simulink model "Prelab1a_simulink_starter"  (R2016a)
settings: Solver=FixedStepDiscrete  StartTime=0.0  StopTime=10.0  FixedStep=5e-3  RelTol=1e-3
settings Model: Creator=katiebyl  LastModifiedBy=katiebyl
settings RTWCC: BuildConfiguration=Faster Runs

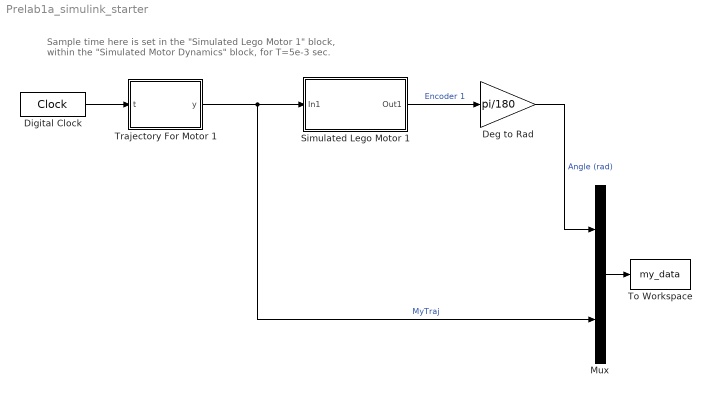
== system Prelab1a_simulink_starter ==
  note: Sample time here is set in the "Simulated Lego Motor 1" block,
      | within the "Simulated Motor Dynamics" block, for T=5e-3 sec.
  Deg to Rad : Gain  Gain=pi/180
  Digital Clock : DigitalClock  SampleTime=5e-3
  Mux : Mux  Inputs=2
  Simulated Lego Motor 1 : Subsystem
  To Workspace : ToWorkspace  VariableName=my_data  SaveFormat=Structure With Time  SampleTime=-1
  Trajectory For Motor 1 : MATLAB Function  TreatAsAtomicUnit=on
  wires:
  Simulated Lego Motor 1/1(Out1) -> Deg to Rad/1  "Encoder 1"
  Deg to Rad/1 -> Mux/1  "Angle (rad)"
  Mux/1 -> To Workspace/1
  Digital Clock/1 -> Trajectory For Motor 1/1(t)
  Trajectory For Motor 1/1(y) -> Mux/2, Simulated Lego Motor 1/1(In1)  "MyTraj"

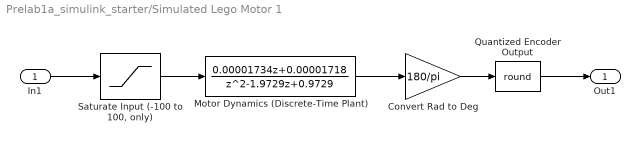
== system Prelab1a_simulink_starter/Simulated Lego Motor 1 ==
  In1 : Inport
  Convert Rad to Deg : Gain  Gain=180/pi
  Motor Dynamics (Discrete-Time Plant) : DiscreteTransferFcn  Numerator="[0.00001734  0.00001718]"  Denominator="[1   -1.9729    0.9729]"
  Quantized Encoder Output : Rounding  Operator=round
  "Saturate Input (-100 to 100, only)" : Saturate  UpperLimit=100  LowerLimit=-100
  Out1 : Outport
  wires:
  In1/1 -> "Saturate Input (-100 to 100, only)"/1
  "Saturate Input (-100 to 100, only)"/1 -> Motor Dynamics (Discrete-Time Plant)/1
  Convert Rad to Deg/1 -> Quantized Encoder Output/1
  Motor Dynamics (Discrete-Time Plant)/1 -> Convert Rad to Deg/1
  Quantized Encoder Output/1 -> Out1/1

== matlab function Prelab1a_simulink_starter/Trajectory For Motor 1 ==
  data: t input; y output
function y = MyTrajectory(t)

%% Define y(t) as a desired TRAJECTORY as a function of TIME

if 1
    %% Example 1: a step, which starts at t=1 second
    t_start = 1; % have the step occur at t = t_start
    StepMag = 100; % For a step in RAW INPUT to motor (open loop)
    % StepMag = 0.3; % for a step in RADIANS, as a TRAJECTORY (closed loop)
    % Here, this the VALUE TO THE MOTOR (analogous to open-loop voltage)
    if t>=t_start
        y = StepMag;
    else
        y = 0;
    end
    
    
elseif 0
    %% Example 2: a trajectory, in RADIANS, for the motor to follow
    t_start = 1;
    A = 0.3; % In RADIANS
    w = 2*2*pi;
    if t>=t_start
        t_use = t - t_start;
        y = A * sin(w*t_use);
    else
        y = 0;
    end
    
elseif 0
    %% Example 3: using interp1() and some waypoints
    ti = [0 1 2 3 100];
    yi = [0 0 20 -30 -30]*(pi/180);
    y = interp1(ti,yi,t);  % LINEAR INTERPOLATION, as a REFERENCE
else
    %% Example 4: using half-cosine function, for smooth transitions
    ypts = [0 0 30 -20 0 0]*pi/180;
    tpts = [0 1 2 3 4 10];
    if t < tpts(2)
        y1 = ypts(1); y2 = ypts(2);
        t1 = tpts(1); t2 = tpts(2);
    elseif t < tpts(3)
        y1 = ypts(2); y2 = ypts(3);
        t1 = tpts(2); t2 = tpts(3);
    elseif t < tpts(4)
        y1 = ypts(3); y2 = ypts(4);
        t1 = tpts(3); t2 = tpts(4);
    elseif t < tpts(5)
        y1 = ypts(4); y2 = ypts(5); % Hold at SAME VALUE
        t1 = tpts(4); t2 = tpts(5);
    else
        y1 = ypts(5); y2 = ypts(6);
        t1 = tpts(5); t2 = tpts(6);
    end
    tPhase = (t-t1) / (t2-t1);  % goes from 0 to 1
    cosVal = cos(pi * tPhase);  % cos(pi*tPhase) will go from 1 to -1...
    y = y1 + (y2 - y1) * (.5 * (1-cosVal)); % cosine shape, going
    % from 0 to 1, as tPhase goes from 0 to pi.
end
